simulink model "TractionEmotorSoftwareArch_DataBus"  (R2026a)
settings: Solver=FixedStepDiscrete
settings Model: DataDictionary=TractionEmotorSoftwareArchInterfaceData.sldd  EnableAccessToBaseWorkspace=off  OrderFunctionsByDependency=on  Creator=dakaihu  LastModifiedBy=dakaihu

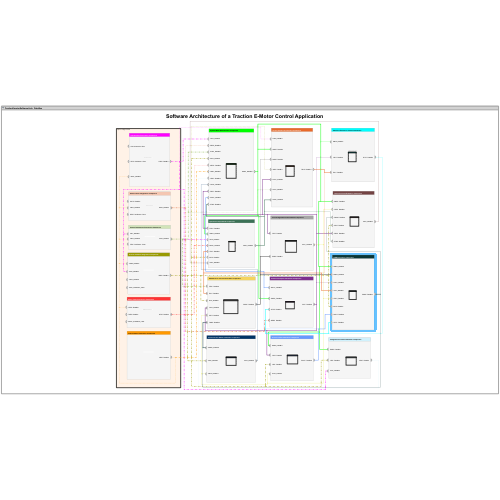
[thumbnail: Simulink's stored preview of the top-level diagram]
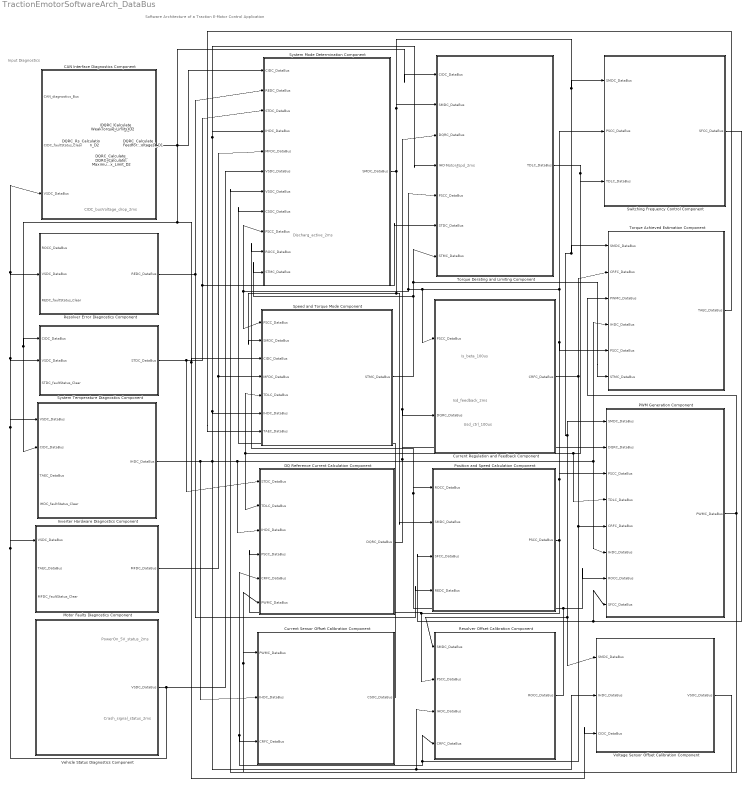
== system TractionEmotorSoftwareArch_DataBus ==
  note: Motor_spd_2ms
  note: Crash_signal_status_2ms
  note: PowerOn_5V_status_2ms
  note: Discharg_active_2ms
  note: Usd_ctrl_100us
  note: Isd_feedback_2ms
  note: Is_beta_100us
  note: CIDC_busVoltage_drop_2ms
  note: Input Diagnostics
  note: Software Architecture of a Traction E-Motor Control Application
  DQRC_Calculate_Feedforward_Voltages _D1 : Inport  OutputFunctionCall=on
  DQRC_Calculate_Optimal_Flux_D1 : Inport  Port=2  OutputFunctionCall=on
  DQRC_Flux_Weakening_Control_D1 : Inport  Port=3  OutputFunctionCall=on
  DQRC_Rs_Calculation_D2 : Inport  Port=4  OutputFunctionCall=on
  DQRC_Calculate_Maximum_Flux_Limit_D2 : Inport  Port=5  OutputFunctionCall=on
  DQRC_Calculate_Torque_Limits_D2 : Inport  Port=6  OutputFunctionCall=on
  CAN Interface Diagnostics Component : Subsystem
      settings: PortSchema="{\"entries\":[{\"content\":{\"headerSize\":26,\"margin\":15,\"minimumSpacing\":25,\"sides\":[{\"content\":{\"connectorIds\":[\"In2\",\"In1\",\"In3\"]},\"type\":\"ConnectorPlacement.EquallySpacedRectSide\",\"uuid\":\"3a2e990d-2ce1-4c6a-a08e-49004fced93c\"},{\"content\":{\"connectorIds\":[\"Out1\"],\"side\":\"RIGHT\"},\"type\":\"ConnectorPlacement.EquallySpacedRectSide\",\"uuid\":\"2e4f52de-0426-461f-b804-44573dbe364d\"},{\"content\":{\"connectorIds\":[],\"side\":\"TOP\"},\"type\":\"ConnectorPlacement.EquallySpacedRectSide\",\"uuid\":\"accbd54d-36a1-4bba-b227-ea03e90f0849\"}]},\"type\":\"ConnectorPlacement.EquallySpacedConnector\",\"uuid\":\"703f56ad-5037-4d99-b3d7-1bfb32b6a309\"}],\"packageUris\":[\"http://schema.mathworks.com/mf0/Connector/R2020b\"],\"version\":\"1.0\"}"
  "Current Regulation and Feedback Component " : Subsystem
      settings: PortSchema="{\"entries\":[{\"content\":{\"headerSize\":26,\"margin\":15,\"minimumSpacing\":25,\"sides\":[{\"content\":{\"connectorIds\":[\"In1\",\"In2\"]},\"type\":\"ConnectorPlacement.EquallySpacedRectSide\",\"uuid\":\"a71464e4-ef65-4500-8253-61f4bcbf30c4\"},{\"content\":{\"connectorIds\":[\"Out1\"],\"side\":\"RIGHT\"},\"type\":\"ConnectorPlacement.EquallySpacedRectSide\",\"uuid\":\"1bcf2d4f-45fa-4d52-8581-70b7b3dbffa8\"},{\"content\":{\"connectorIds\":[],\"side\":\"TOP\"},\"type\":\"ConnectorPlacement.EquallySpacedRectSide\",\"uuid\":\"1184bab8-6b51-4118-818c-c187fd989a95\"},{\"content\":{\"connectorIds\":[],\"side\":\"HIDDEN\"},\"type\":\"ConnectorPlacement.EquallySpacedRectSide\",\"uuid\":\"65ee186c-6391-47f9-9292-b3d987265f69\"}]},\"type\":\"ConnectorPlacement.EquallySpacedConnector\",\"uuid\":\"052954ad-d64a-4fb3-8bba-30843ae03591\"}],\"packageUris\":[\"http://schema.mathworks.com/mf0/Connector/R2020b\"],\"version\":\"1.0\"}"
  "Current Sensor Offset Calibration Component " : Subsystem
      settings: PortSchema="{\"entries\":[{\"content\":{\"headerSize\":26,\"margin\":15,\"minimumSpacing\":25,\"sides\":[{\"content\":{\"connectorIds\":[\"In1\",\"In2\",\"In3\"]},\"type\":\"ConnectorPlacement.EquallySpacedRectSide\",\"uuid\":\"a71464e4-ef65-4500-8253-61f4bcbf30c4\"},{\"content\":{\"connectorIds\":[\"Out1\"],\"side\":\"RIGHT\"},\"type\":\"ConnectorPlacement.EquallySpacedRectSide\",\"uuid\":\"1bcf2d4f-45fa-4d52-8581-70b7b3dbffa8\"},{\"content\":{\"connectorIds\":[],\"side\":\"TOP\"},\"type\":\"ConnectorPlacement.EquallySpacedRectSide\",\"uuid\":\"1184bab8-6b51-4118-818c-c187fd989a95\"},{\"content\":{\"connectorIds\":[],\"side\":\"HIDDEN\"},\"type\":\"ConnectorPlacement.EquallySpacedRectSide\",\"uuid\":\"65ee186c-6391-47f9-9292-b3d987265f69\"}]},\"type\":\"ConnectorPlacement.EquallySpacedConnector\",\"uuid\":\"052954ad-d64a-4fb3-8bba-30843ae03591\"}],\"packageUris\":[\"http://schema.mathworks.com/mf0/Connector/R2020b\"],\"version\":\"1.0\"}"
  DQ Reference Current Calculation Component : Subsystem
      settings: PortSchema="{\"entries\":[{\"content\":{\"headerSize\":26,\"margin\":15,\"minimumSpacing\":25,\"sides\":[{\"content\":{\"connectorIds\":[\"In1\",\"In2\",\"In6\",\"In3\",\"In4\",\"In5\"]},\"type\":\"ConnectorPlacement.EquallySpacedRectSide\",\"uuid\":\"a71464e4-ef65-4500-8253-61f4bcbf30c4\"},{\"content\":{\"connectorIds\":[\"Out1\"],\"side\":\"RIGHT\"},\"type\":\"ConnectorPlacement.EquallySpacedRectSide\",\"uuid\":\"1bcf2d4f-45fa-4d52-8581-70b7b3dbffa8\"},{\"content\":{\"connectorIds\":[],\"side\":\"TOP\"},\"type\":\"ConnectorPlacement.EquallySpacedRectSide\",\"uuid\":\"1184bab8-6b51-4118-818c-c187fd989a95\"},{\"content\":{\"connectorIds\":[],\"side\":\"HIDDEN\"},\"type\":\"ConnectorPlacement.EquallySpacedRectSide\",\"uuid\":\"65ee186c-6391-47f9-9292-b3d987265f69\"}]},\"type\":\"ConnectorPlacement.EquallySpacedConnector\",\"uuid\":\"052954ad-d64a-4fb3-8bba-30843ae03591\"}],\"packageUris\":[\"http://schema.mathworks.com/mf0/Connector/R2020b\"],\"version\":\"1.0\"}"
  Inverter Hardware Diagnostics Component : Subsystem
      settings: PortSchema="{\"entries\":[{\"content\":{\"headerSize\":26,\"margin\":15,\"minimumSpacing\":25,\"sides\":[{\"content\":{\"connectorIds\":[\"In1\",\"In2\",\"In3\",\"In4\"]},\"type\":\"ConnectorPlacement.EquallySpacedRectSide\",\"uuid\":\"3a2e990d-2ce1-4c6a-a08e-49004fced93c\"},{\"content\":{\"connectorIds\":[\"Out1\"],\"side\":\"RIGHT\"},\"type\":\"ConnectorPlacement.EquallySpacedRectSide\",\"uuid\":\"2e4f52de-0426-461f-b804-44573dbe364d\"},{\"content\":{\"connectorIds\":[],\"side\":\"TOP\"},\"type\":\"ConnectorPlacement.EquallySpacedRectSide\",\"uuid\":\"accbd54d-36a1-4bba-b227-ea03e90f0849\"}]},\"type\":\"ConnectorPlacement.EquallySpacedConnector\",\"uuid\":\"703f56ad-5037-4d99-b3d7-1bfb32b6a309\"}],\"packageUris\":[\"http://schema.mathworks.com/mf0/Connector/R2020b\"],\"version\":\"1.0\"}"
  Motor Faults Diagnostics Component : Subsystem
      settings: PortSchema="{\"entries\":[{\"content\":{\"headerSize\":26,\"margin\":15,\"minimumSpacing\":25,\"sides\":[{\"content\":{\"connectorIds\":[\"In1\",\"In2\",\"In3\"]},\"type\":\"ConnectorPlacement.EquallySpacedRectSide\",\"uuid\":\"3a2e990d-2ce1-4c6a-a08e-49004fced93c\"},{\"content\":{\"connectorIds\":[\"Out1\"],\"side\":\"RIGHT\"},\"type\":\"ConnectorPlacement.EquallySpacedRectSide\",\"uuid\":\"2e4f52de-0426-461f-b804-44573dbe364d\"},{\"content\":{\"connectorIds\":[],\"side\":\"TOP\"},\"type\":\"ConnectorPlacement.EquallySpacedRectSide\",\"uuid\":\"accbd54d-36a1-4bba-b227-ea03e90f0849\"}]},\"type\":\"ConnectorPlacement.EquallySpacedConnector\",\"uuid\":\"703f56ad-5037-4d99-b3d7-1bfb32b6a309\"}],\"packageUris\":[\"http://schema.mathworks.com/mf0/Connector/R2020b\"],\"version\":\"1.0\"}"
  PWM Generation Component : Subsystem
      settings: PortSchema="{\"entries\":[{\"content\":{\"headerSize\":26,\"margin\":15,\"minimumSpacing\":25,\"sides\":[{\"content\":{\"connectorIds\":[\"In2\",\"In1\",\"In3\",\"In4\",\"In6\",\"In7\",\"In8\",\"In5\"]},\"type\":\"ConnectorPlacement.EquallySpacedRectSide\",\"uuid\":\"a71464e4-ef65-4500-8253-61f4bcbf30c4\"},{\"content\":{\"connectorIds\":[\"Out1\"],\"side\":\"RIGHT\"},\"type\":\"ConnectorPlacement.EquallySpacedRectSide\",\"uuid\":\"1bcf2d4f-45fa-4d52-8581-70b7b3dbffa8\"},{\"content\":{\"connectorIds\":[],\"side\":\"TOP\"},\"type\":\"ConnectorPlacement.EquallySpacedRectSide\",\"uuid\":\"1184bab8-6b51-4118-818c-c187fd989a95\"},{\"content\":{\"connectorIds\":[],\"side\":\"HIDDEN\"},\"type\":\"ConnectorPlacement.EquallySpacedRectSide\",\"uuid\":\"65ee186c-6391-47f9-9292-b3d987265f69\"}]},\"type\":\"ConnectorPlacement.EquallySpacedConnector\",\"uuid\":\"052954ad-d64a-4fb3-8bba-30843ae03591\"}],\"packageUris\":[\"http://schema.mathworks.com/mf0/Connector/R2020b\"],\"version\":\"1.0\"}"
  Position and Speed Calculation Component : Subsystem
      settings: PortSchema="{\"entries\":[{\"content\":{\"headerSize\":26,\"margin\":15,\"minimumSpacing\":25,\"sides\":[{\"content\":{\"connectorIds\":[\"In1\",\"In2\",\"In3\",\"In4\"]},\"type\":\"ConnectorPlacement.EquallySpacedRectSide\",\"uuid\":\"a71464e4-ef65-4500-8253-61f4bcbf30c4\"},{\"content\":{\"connectorIds\":[\"Out1\"],\"side\":\"RIGHT\"},\"type\":\"ConnectorPlacement.EquallySpacedRectSide\",\"uuid\":\"1bcf2d4f-45fa-4d52-8581-70b7b3dbffa8\"},{\"content\":{\"connectorIds\":[],\"side\":\"TOP\"},\"type\":\"ConnectorPlacement.EquallySpacedRectSide\",\"uuid\":\"1184bab8-6b51-4118-818c-c187fd989a95\"},{\"content\":{\"connectorIds\":[],\"side\":\"HIDDEN\"},\"type\":\"ConnectorPlacement.EquallySpacedRectSide\",\"uuid\":\"65ee186c-6391-47f9-9292-b3d987265f69\"}]},\"type\":\"ConnectorPlacement.EquallySpacedConnector\",\"uuid\":\"052954ad-d64a-4fb3-8bba-30843ae03591\"}],\"packageUris\":[\"http://schema.mathworks.com/mf0/Connector/R2020b\"],\"version\":\"1.0\"}"
  Resolver Error Diagnostics Component : Subsystem
      settings: PortSchema="{\"entries\":[{\"content\":{\"headerSize\":26,\"margin\":15,\"minimumSpacing\":25,\"sides\":[{\"content\":{\"connectorIds\":[\"In1\",\"In2\",\"In3\"]},\"type\":\"ConnectorPlacement.EquallySpacedRectSide\",\"uuid\":\"3a2e990d-2ce1-4c6a-a08e-49004fced93c\"},{\"content\":{\"connectorIds\":[\"Out1\"],\"side\":\"RIGHT\"},\"type\":\"ConnectorPlacement.EquallySpacedRectSide\",\"uuid\":\"2e4f52de-0426-461f-b804-44573dbe364d\"},{\"content\":{\"side\":\"TOP\"},\"type\":\"ConnectorPlacement.EquallySpacedRectSide\",\"uuid\":\"accbd54d-36a1-4bba-b227-ea03e90f0849\"}]},\"type\":\"ConnectorPlacement.EquallySpacedConnector\",\"uuid\":\"703f56ad-5037-4d99-b3d7-1bfb32b6a309\"}],\"packageUris\":[\"http://schema.mathworks.com/mf0/Connector/R2020b\"],\"version\":\"1.0\"}"
  "Resolver Offset Calibration Component " : Subsystem
      settings: PortSchema="{\"entries\":[{\"content\":{\"headerSize\":26,\"margin\":15,\"minimumSpacing\":25,\"sides\":[{\"content\":{\"connectorIds\":[\"In1\",\"In2\",\"In3\",\"In4\"]},\"type\":\"ConnectorPlacement.EquallySpacedRectSide\",\"uuid\":\"b2f30fca-3d8e-46ee-af1d-282b22b9b844\"},{\"content\":{\"connectorIds\":[\"Out1\"],\"side\":\"RIGHT\"},\"type\":\"ConnectorPlacement.EquallySpacedRectSide\",\"uuid\":\"2d7d706d-eac4-4c73-84e8-2a36a393a616\"},{\"content\":{\"connectorIds\":[],\"side\":\"TOP\"},\"type\":\"ConnectorPlacement.EquallySpacedRectSide\",\"uuid\":\"b52ae510-b7cc-4ed0-8d34-4a095deae41b\"}]},\"type\":\"ConnectorPlacement.EquallySpacedConnector\",\"uuid\":\"1257e7cc-1858-4bc4-ab05-7b00060cf0d5\"}],\"packageUris\":[\"http://schema.mathworks.com/mf0/Connector/R2020b\"],\"version\":\"1.0\"}"
  Speed and Torque Mode Component : Subsystem
      settings: PortSchema="{\"entries\":[{\"content\":{\"headerSize\":26,\"margin\":15,\"minimumSpacing\":25,\"sides\":[{\"content\":{\"connectorIds\":[\"In4\",\"In1\",\"In2\",\"In3\",\"In5\",\"In7\",\"In6\"]},\"type\":\"ConnectorPlacement.EquallySpacedRectSide\",\"uuid\":\"a71464e4-ef65-4500-8253-61f4bcbf30c4\"},{\"content\":{\"connectorIds\":[\"Out1\"],\"side\":\"RIGHT\"},\"type\":\"ConnectorPlacement.EquallySpacedRectSide\",\"uuid\":\"1bcf2d4f-45fa-4d52-8581-70b7b3dbffa8\"},{\"content\":{\"connectorIds\":[],\"side\":\"TOP\"},\"type\":\"ConnectorPlacement.EquallySpacedRectSide\",\"uuid\":\"1184bab8-6b51-4118-818c-c187fd989a95\"},{\"content\":{\"connectorIds\":[],\"side\":\"HIDDEN\"},\"type\":\"ConnectorPlacement.EquallySpacedRectSide\",\"uuid\":\"65ee186c-6391-47f9-9292-b3d987265f69\"}]},\"type\":\"ConnectorPlacement.EquallySpacedConnector\",\"uuid\":\"052954ad-d64a-4fb3-8bba-30843ae03591\"}],\"packageUris\":[\"http://schema.mathworks.com/mf0/Connector/R2020b\"],\"version\":\"1.0\"}"
  Switching Frequency Control Component : Subsystem
      settings: PortSchema="{\"entries\":[{\"content\":{\"headerSize\":26,\"margin\":15,\"minimumSpacing\":25,\"sides\":[{\"content\":{\"connectorIds\":[\"In1\",\"In2\",\"In3\"]},\"type\":\"ConnectorPlacement.EquallySpacedRectSide\",\"uuid\":\"a71464e4-ef65-4500-8253-61f4bcbf30c4\"},{\"content\":{\"connectorIds\":[\"Out1\"],\"side\":\"RIGHT\"},\"type\":\"ConnectorPlacement.EquallySpacedRectSide\",\"uuid\":\"1bcf2d4f-45fa-4d52-8581-70b7b3dbffa8\"},{\"content\":{\"connectorIds\":[],\"side\":\"TOP\"},\"type\":\"ConnectorPlacement.EquallySpacedRectSide\",\"uuid\":\"1184bab8-6b51-4118-818c-c187fd989a95\"},{\"content\":{\"connectorIds\":[],\"side\":\"HIDDEN\"},\"type\":\"ConnectorPlacement.EquallySpacedRectSide\",\"uuid\":\"65ee186c-6391-47f9-9292-b3d987265f69\"}]},\"type\":\"ConnectorPlacement.EquallySpacedConnector\",\"uuid\":\"052954ad-d64a-4fb3-8bba-30843ae03591\"}],\"packageUris\":[\"http://schema.mathworks.com/mf0/Connector/R2020b\"],\"version\":\"1.0\"}"
  "System Mode Determination Component " : Subsystem
      settings: PortSchema="{\"entries\":[{\"content\":{\"headerSize\":26,\"margin\":15,\"minimumSpacing\":25,\"sides\":[{\"content\":{\"connectorIds\":[\"In1\",\"In2\",\"In3\",\"In4\",\"In5\",\"In6\",\"In9\",\"In8\",\"In10\",\"In7\",\"In11\"]},\"type\":\"ConnectorPlacement.EquallySpacedRectSide\",\"uuid\":\"a71464e4-ef65-4500-8253-61f4bcbf30c4\"},{\"content\":{\"connectorIds\":[\"Out1\"],\"side\":\"RIGHT\"},\"type\":\"ConnectorPlacement.EquallySpacedRectSide\",\"uuid\":\"1bcf2d4f-45fa-4d52-8581-70b7b3dbffa8\"},{\"content\":{\"connectorIds\":[],\"side\":\"TOP\"},\"type\":\"ConnectorPlacement.EquallySpacedRectSide\",\"uuid\":\"1184bab8-6b51-4118-818c-c187fd989a95\"},{\"content\":{\"connectorIds\":[],\"side\":\"BOTTOM\"},\"type\":\"ConnectorPlacement.EquallySpacedRectSide\",\"uuid\":\"db64044a-7d50-4610-bfd1-d03b668d605f\"},{\"content\":{\"connectorIds\":[],\"side\":\"HIDDEN\"},\"type\":\"ConnectorPlacement.EquallySpacedRectSide\",\"uuid\":\"65ee186c-6391-47f9-9292-b3d987265f69\"}]},\"type\":\"ConnectorPlacement.EquallySpacedConnector\",\"uuid\":\"052954ad-d64a-4fb3-8bba-30843ae03591\"}],\"packageUris\":[\"http://schema.mathworks.com/mf0/Connector/R2020b\"],\"version\":\"1.0\"}"
  System Temperature Diagnostics Component : Subsystem
      settings: PortSchema="{\"entries\":[{\"content\":{\"headerSize\":26,\"margin\":15,\"minimumSpacing\":25,\"sides\":[{\"content\":{\"connectorIds\":[\"In1\",\"In2\",\"In3\"]},\"type\":\"ConnectorPlacement.EquallySpacedRectSide\",\"uuid\":\"3a2e990d-2ce1-4c6a-a08e-49004fced93c\"},{\"content\":{\"connectorIds\":[\"Out1\"],\"side\":\"RIGHT\"},\"type\":\"ConnectorPlacement.EquallySpacedRectSide\",\"uuid\":\"2e4f52de-0426-461f-b804-44573dbe364d\"},{\"content\":{\"connectorIds\":[],\"side\":\"TOP\"},\"type\":\"ConnectorPlacement.EquallySpacedRectSide\",\"uuid\":\"accbd54d-36a1-4bba-b227-ea03e90f0849\"}]},\"type\":\"ConnectorPlacement.EquallySpacedConnector\",\"uuid\":\"703f56ad-5037-4d99-b3d7-1bfb32b6a309\"}],\"packageUris\":[\"http://schema.mathworks.com/mf0/Connector/R2020b\"],\"version\":\"1.0\"}"
  Torque Achieved Estimation Component : Subsystem
      settings: PortSchema="{\"entries\":[{\"content\":{\"headerSize\":26,\"margin\":15,\"minimumSpacing\":25,\"sides\":[{\"content\":{\"connectorIds\":[\"In1\",\"In2\",\"In3\",\"In4\",\"In5\",\"In6\"]},\"type\":\"ConnectorPlacement.EquallySpacedRectSide\",\"uuid\":\"a71464e4-ef65-4500-8253-61f4bcbf30c4\"},{\"content\":{\"connectorIds\":[\"Out1\"],\"side\":\"RIGHT\"},\"type\":\"ConnectorPlacement.EquallySpacedRectSide\",\"uuid\":\"1bcf2d4f-45fa-4d52-8581-70b7b3dbffa8\"},{\"content\":{\"connectorIds\":[],\"side\":\"TOP\"},\"type\":\"ConnectorPlacement.EquallySpacedRectSide\",\"uuid\":\"1184bab8-6b51-4118-818c-c187fd989a95\"},{\"content\":{\"connectorIds\":[],\"side\":\"HIDDEN\"},\"type\":\"ConnectorPlacement.EquallySpacedRectSide\",\"uuid\":\"65ee186c-6391-47f9-9292-b3d987265f69\"}]},\"type\":\"ConnectorPlacement.EquallySpacedConnector\",\"uuid\":\"052954ad-d64a-4fb3-8bba-30843ae03591\"}],\"packageUris\":[\"http://schema.mathworks.com/mf0/Connector/R2020b\"],\"version\":\"1.0\"}"
  Torque Derating and Limiting Component : Subsystem
      settings: PortSchema="{\"entries\":[{\"content\":{\"headerSize\":26,\"margin\":15,\"minimumSpacing\":25,\"sides\":[{\"content\":{\"connectorIds\":[\"In5\",\"In1\",\"In2\",\"In3\",\"In4\",\"In6\",\"In7\"]},\"type\":\"ConnectorPlacement.EquallySpacedRectSide\",\"uuid\":\"fd31d295-2ee8-4010-a085-72a956fb88db\"},{\"content\":{\"connectorIds\":[\"Out1\"],\"side\":\"RIGHT\"},\"type\":\"ConnectorPlacement.EquallySpacedRectSide\",\"uuid\":\"6e15e65a-8b2c-4657-b6d9-6871ed377dcc\"},{\"content\":{\"connectorIds\":[],\"side\":\"TOP\"},\"type\":\"ConnectorPlacement.EquallySpacedRectSide\",\"uuid\":\"e10f5a11-10a3-425e-91ff-fff14d159c09\"},{\"content\":{\"connectorIds\":[],\"side\":\"BOTTOM\"},\"type\":\"ConnectorPlacement.EquallySpacedRectSide\",\"uuid\":\"618ca321-1f5f-4aa6-a247-3a346143f509\"}]},\"type\":\"ConnectorPlacement.EquallySpacedConnector\",\"uuid\":\"062b7cf1-4df3-4671-ab85-e62a20780700\"}],\"packageUris\":[\"http://schema.mathworks.com/mf0/Connector/R2020b\"],\"version\":\"1.0\"}"
  Vehicle Status Diagnostics Component : Subsystem
      settings: PortSchema="{\"entries\":[{\"content\":{\"headerSize\":26,\"margin\":15,\"minimumSpacing\":25,\"sides\":[{\"content\":{\"connectorIds\":[]},\"type\":\"ConnectorPlacement.EquallySpacedRectSide\",\"uuid\":\"3a2e990d-2ce1-4c6a-a08e-49004fced93c\"},{\"content\":{\"connectorIds\":[\"Out1\"],\"side\":\"RIGHT\"},\"type\":\"ConnectorPlacement.EquallySpacedRectSide\",\"uuid\":\"2e4f52de-0426-461f-b804-44573dbe364d\"},{\"content\":{\"connectorIds\":[],\"side\":\"TOP\"},\"type\":\"ConnectorPlacement.EquallySpacedRectSide\",\"uuid\":\"accbd54d-36a1-4bba-b227-ea03e90f0849\"}]},\"type\":\"ConnectorPlacement.EquallySpacedConnector\",\"uuid\":\"703f56ad-5037-4d99-b3d7-1bfb32b6a309\"}],\"packageUris\":[\"http://schema.mathworks.com/mf0/Connector/R2020b\"],\"version\":\"1.0\"}"
  Voltage Sensor Offset Calibration Component : Subsystem
      settings: PortSchema="{\"entries\":[{\"content\":{\"headerSize\":26,\"margin\":15,\"minimumSpacing\":25,\"sides\":[{\"content\":{\"connectorIds\":[\"In1\",\"In3\",\"In2\"]},\"type\":\"ConnectorPlacement.EquallySpacedRectSide\",\"uuid\":\"a71464e4-ef65-4500-8253-61f4bcbf30c4\"},{\"content\":{\"connectorIds\":[\"Out1\"],\"side\":\"RIGHT\"},\"type\":\"ConnectorPlacement.EquallySpacedRectSide\",\"uuid\":\"1bcf2d4f-45fa-4d52-8581-70b7b3dbffa8\"},{\"content\":{\"connectorIds\":[],\"side\":\"TOP\"},\"type\":\"ConnectorPlacement.EquallySpacedRectSide\",\"uuid\":\"1184bab8-6b51-4118-818c-c187fd989a95\"},{\"content\":{\"connectorIds\":[],\"side\":\"HIDDEN\"},\"type\":\"ConnectorPlacement.EquallySpacedRectSide\",\"uuid\":\"65ee186c-6391-47f9-9292-b3d987265f69\"}]},\"type\":\"ConnectorPlacement.EquallySpacedConnector\",\"uuid\":\"052954ad-d64a-4fb3-8bba-30843ae03591\"}],\"packageUris\":[\"http://schema.mathworks.com/mf0/Connector/R2020b\"],\"version\":\"1.0\"}"
  wires:
  Resolver Error Diagnostics Component/1(REDC_DataBus) -> "System Mode Determination Component "/2(REDC_DataBus), Position and Speed Calculation Component/4(REDC_DataBus)
  System Temperature Diagnostics Component/1(STDC_DataBus) -> DQ Reference Current Calculation Component/1(STDC_DataBus), Torque Derating and Limiting Component/6(STDC_DataBus), "System Mode Determination Component "/3(STDC_DataBus)
  Inverter Hardware Diagnostics Component/1(IHDC_DataBus) -> "Current Sensor Offset Calibration Component "/2(IHDC_DataBus), PWM Generation Component/7(IHDC_DataBus), Torque Achieved Estimation Component/4(IHDC_DataBus), DQ Reference Current Calculation Component/6(IHDC_DataBus), "Resolver Offset Calibration Component "/3(IHDC_DataBus), Voltage Sensor Offset Calibration Component/3(IHDC_DataBus), "System Mode Determination Component "/4(IHDC_DataBus), Torque Derating and Limiting Component/3(IHDC_DataBus), Speed and Torque Mode Component/7(IHDC_DataBus)
  Motor Faults Diagnostics Component/1(MFDC_DataBus) -> "System Mode Determination Component "/5(MFDC_DataBus), Speed and Torque Mode Component/3(MFDC_DataBus)
  Vehicle Status Diagnostics Component/1(VSDC_DataBus) -> "System Mode Determination Component "/6(VSDC_DataBus), Motor Faults Diagnostics Component/1(VSDC_DataBus), System Temperature Diagnostics Component/2(VSDC_DataBus), Resolver Error Diagnostics Component/2(VSDC_DataBus), CAN Interface Diagnostics Component/3(VSDC_DataBus), Inverter Hardware Diagnostics Component/1(VSDC_DataBus)
  "System Mode Determination Component "/1(SMDC_DataBus) -> Position and Speed Calculation Component/2(SMDC_DataBus), Speed and Torque Mode Component/1(SMDC_DataBus), Torque Derating and Limiting Component/1(SMDC_DataBus), PWM Generation Component/2(SMDC_DataBus), Voltage Sensor Offset Calibration Component/1(SMDC_DataBus), "Resolver Offset Calibration Component "/1(SMDC_DataBus), Torque Achieved Estimation Component/1(SMDC_DataBus), Switching Frequency Control Component/1(SMDC_DataBus)
  "Resolver Offset Calibration Component "/1(ROCC_DataBus) -> "System Mode Determination Component "/7(ROCC_DataBus), Position and Speed Calculation Component/1(ROCC_DataBus), PWM Generation Component/8(ROCC_DataBus)
  "Current Sensor Offset Calibration Component "/1(CSOC_DataBus) -> "System Mode Determination Component "/8(CSOC_DataBus)
  Voltage Sensor Offset Calibration Component/1(VSOC_DataBus) -> "System Mode Determination Component "/9(VSOC_DataBus)
  Position and Speed Calculation Component/1(PSCC_DataBus) -> Torque Achieved Estimation Component/5(PSCC_DataBus), "Current Regulation and Feedback Component "/1(PSCC_DataBus), Torque Derating and Limiting Component/4(PSCC_DataBus), Speed and Torque Mode Component/4(PSCC_DataBus), "System Mode Determination Component "/10(PSCC_DataBus), Switching Frequency Control Component/2(PSCC_DataBus), PWM Generation Component/3(PSCC_DataBus), "Resolver Offset Calibration Component "/2(PSCC_DataBus), DQ Reference Current Calculation Component/3(PSCC_DataBus)
  Speed and Torque Mode Component/1(STMC_DataBus) -> Torque Achieved Estimation Component/6(STMC_DataBus), Torque Derating and Limiting Component/7(STMC_DataBus), "System Mode Determination Component "/11(STMC_DataBus)
  DQ Reference Current Calculation Component/1(DQRC_DataBus) -> Torque Derating and Limiting Component/2(DQRC_DataBus), "Current Regulation and Feedback Component "/2(DQRC_DataBus), PWM Generation Component/1(DQRC_DataBus)
  Torque Derating and Limiting Component/1(TDLC_DataBus) -> Switching Frequency Control Component/3(TDLC_DataBus), PWM Generation Component/4(TDLC_DataBus), DQ Reference Current Calculation Component/2(TDLC_DataBus), Speed and Torque Mode Component/5(TDLC_DataBus)
  "Current Regulation and Feedback Component "/1(CRFC_DataBus) -> Torque Achieved Estimation Component/2(CRFC_DataBus), "Resolver Offset Calibration Component "/4(CRFC_DataBus), "Current Sensor Offset Calibration Component "/3(CRFC_DataBus), DQ Reference Current Calculation Component/4(CRFC_DataBus), PWM Generation Component/6(CRFC_DataBus)
  PWM Generation Component/1(PWMC_DataBus) -> DQ Reference Current Calculation Component/5(PWMC_DataBus), "Current Sensor Offset Calibration Component "/1(PWMC_DataBus), Torque Achieved Estimation Component/3(PWMC_DataBus)
  Switching Frequency Control Component/1(SFCC_DataBus) -> Position and Speed Calculation Component/3(SFCC_DataBus), PWM Generation Component/5(SFCC_DataBus)
  Torque Achieved Estimation Component/1(TAEC_DataBus) -> Speed and Torque Mode Component/6(TAEC_DataBus)
  CAN Interface Diagnostics Component/1(CIDC_DataBus) -> "System Mode Determination Component "/1(CIDC_DataBus), Speed and Torque Mode Component/2(CIDC_DataBus), Voltage Sensor Offset Calibration Component/2(CIDC_DataBus), Inverter Hardware Diagnostics Component/2(CIDC_DataBus), System Temperature Diagnostics Component/1(CIDC_DataBus), Torque Derating and Limiting Component/5(CIDC_DataBus)

== system TractionEmotorSoftwareArch_DataBus/CAN Interface Diagnostics Component ==
  note: CIDC: CAN Interface Diagnostics Component
  Bus Element In1 : Inport  PortName=CIDC_faultStatus_Clear
  Bus Element In2 : Inport  Port=2  PortName=CAN_diagnostics_Bus
  Bus Element In3 : Inport  Port=3  PortName=VSDC_DataBus
  Bus Element Out8 : Outport  PortName=CIDC_DataBus

== system TractionEmotorSoftwareArch_DataBus/Current Regulation and Feedback Component  ==
  note: CRFC: Currents Regulation and Feedback Component
  Bus Element In1 : Inport  PortName=PSCC_DataBus
  Bus Element In2 : Inport  Port=2  PortName=DQRC_DataBus
  CRFC : ModelReference  ModelNameDialog=CurrentRegulationandFeedbackComponent  SimulationMode=Normal  ScheduleRates=on  ModelReferenceVersion=7.0
      settings: PortSchema="{\"entries\":[{\"content\":{\"headerSize\":38,\"margin\":15,\"minimumSpacing\":25,\"sides\":[{\"content\":{\"connectorIds\":[\"In1\",\"In2\",\"In3\",\"In4\",\"In5\",\"In6\",\"In7\",\"In8\",\"In9\",\"In10\",\"In11\",\"In12\"]},\"type\":\"ConnectorPlacement.EquallySpacedRectSide\",\"uuid\":\"43f14977-22c5-403b-bcbc-53575b3aceee\"},{\"content\":{\"connectorIds\":[\"Out1\",\"Out2\",\"Out3\",\"Out4\",\"Out5\",\"Out6\",\"Out7\",\"Out8\",\"Out9\",\"Out10\",\"Out11\"],\"side\":\"RIGHT\"},\"type\":\"ConnectorPlacement.EquallySpacedRectSide\",\"uuid\":\"d93cf4b9-940c-436a-9f2b-9eb79a050f7a\"},{\"content\":{\"side\":\"TOP\"},\"type\":\"ConnectorPlacement.EquallySpacedRectSide\",\"uuid\":\"b3e7cb9e-f235-4106-b3bb-4ca948939197\"},{\"content\":{\"side\":\"HIDDEN\"},\"type\":\"ConnectorPlacement.EquallySpacedRectSide\",\"uuid\":\"291ccf75-5793-4f13-97ee-51f98f8a6b6f\"}]},\"type\":\"ConnectorPlacement.EquallySpacedConnector\",\"uuid\":\"a3b713dd-1bd4-4226-93ff-27d7db6c05ec\"}],\"packageUris\":[\"http://schema.mathworks.com/mf0/Connector/R2020b\"],\"version\":\"1.0\"}"
  Bus Element Out1 : Outport  PortName=CRFC_DataBus

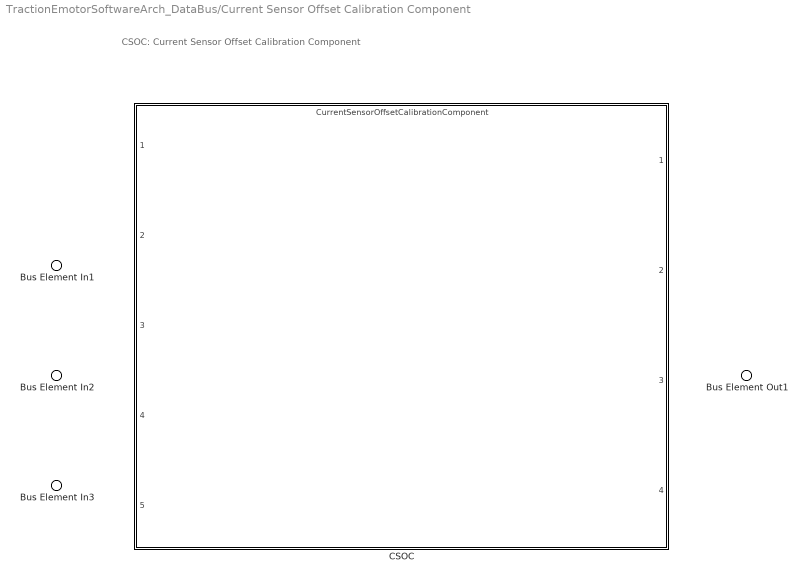
== system TractionEmotorSoftwareArch_DataBus/Current Sensor Offset Calibration Component  ==
  note: CSOC: Current Sensor Offset Calibration Component
  Bus Element In1 : Inport  PortName=PWMC_DataBus
  Bus Element In2 : Inport  Port=2  PortName=IHDC_DataBus
  Bus Element In3 : Inport  Port=3  PortName=CRFC_DataBus
  CSOC : ModelReference  ModelNameDialog=CurrentSensorOffsetCalibrationComponent  SimulationMode=Normal  ScheduleRates=on  ModelReferenceVersion=7.0
      settings: PortSchema="{\"entries\":[{\"content\":{\"headerSize\":38,\"margin\":15,\"minimumSpacing\":25,\"sides\":[{\"content\":{\"connectorIds\":[\"In1\",\"In2\",\"In3\",\"In4\",\"In5\"]},\"type\":\"ConnectorPlacement.EquallySpacedRectSide\",\"uuid\":\"43f14977-22c5-403b-bcbc-53575b3aceee\"},{\"content\":{\"connectorIds\":[\"Out1\",\"Out2\",\"Out3\",\"Out4\"],\"side\":\"RIGHT\"},\"type\":\"ConnectorPlacement.EquallySpacedRectSide\",\"uuid\":\"d93cf4b9-940c-436a-9f2b-9eb79a050f7a\"},{\"content\":{\"side\":\"TOP\"},\"type\":\"ConnectorPlacement.EquallySpacedRectSide\",\"uuid\":\"b3e7cb9e-f235-4106-b3bb-4ca948939197\"},{\"content\":{\"side\":\"HIDDEN\"},\"type\":\"ConnectorPlacement.EquallySpacedRectSide\",\"uuid\":\"d508bc3c-50c4-40a2-9dd3-c5ccc3c4a7e2\"}]},\"type\":\"ConnectorPlacement.EquallySpacedConnector\",\"uuid\":\"a3b713dd-1bd4-4226-93ff-27d7db6c05ec\"}],\"packageUris\":[\"http://schema.mathworks.com/mf0/Connector/R2020b\"],\"version\":\"1.0\"}"
  Bus Element Out1 : Outport  PortName=CSOC_DataBus

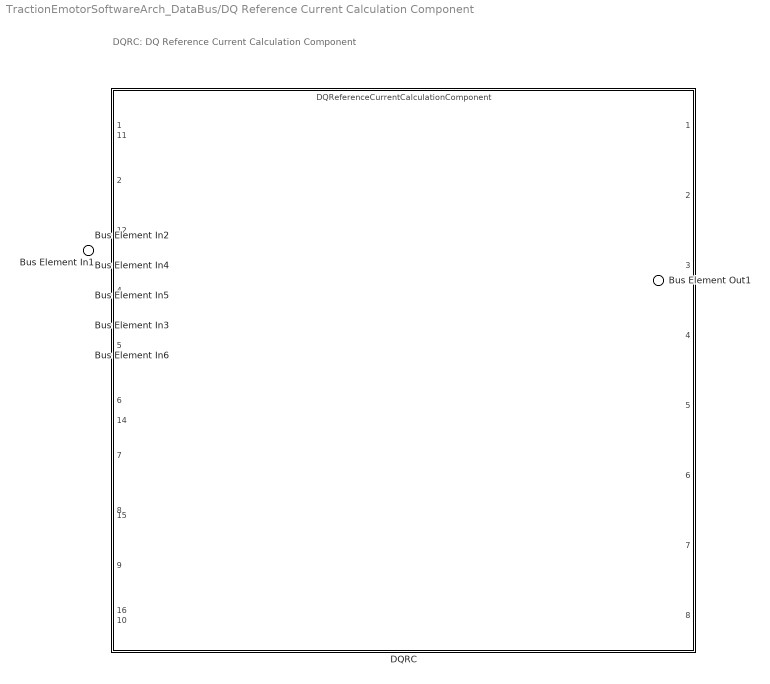
== system TractionEmotorSoftwareArch_DataBus/DQ Reference Current Calculation Component ==
  note: DQRC: DQ Reference Current Calculation Component
  Bus Element In1 : Inport  PortName=STDC_DataBus  Element=STDC_motorTemp_2ms
  Bus Element In2 : Inport  Port=2  PortName=TDLC_DataBus
  Bus Element In4 : Inport  Port=3  PortName=PSCC_DataBus
  Bus Element In5 : Inport  Port=4  PortName=CRFC_DataBus
  Bus Element In3 : Inport  Port=5  PortName=PWMC_DataBus
  Bus Element In6 : Inport  Port=6  PortName=IHDC_DataBus
  DQRC : ModelReference  ModelNameDialog=DQReferenceCurrentCalculationComponent  SimulationMode=Normal  ScheduleRates=on  ModelReferenceVersion=2.3
      settings: PortSchema="{\"entries\":[{\"content\":{\"headerSize\":38,\"margin\":15,\"minimumSpacing\":25,\"sides\":[{\"content\":{\"connectorIds\":[\"In1\",\"In2\",\"In3\",\"In4\",\"In5\",\"In6\",\"In7\",\"In8\",\"In9\",\"In10\"]},\"type\":\"ConnectorPlacement.EquallySpacedRectSide\",\"uuid\":\"43f14977-22c5-403b-bcbc-53575b3aceee\"},{\"content\":{\"connectorIds\":[\"Out1\",\"Out2\",\"Out3\",\"Out4\",\"Out5\",\"Out6\",\"Out7\",\"Out8\"],\"side\":\"RIGHT\"},\"type\":\"ConnectorPlacement.EquallySpacedRectSide\",\"uuid\":\"d93cf4b9-940c-436a-9f2b-9eb79a050f7a\"},{\"content\":{\"side\":\"TOP\"},\"type\":\"ConnectorPlacement.EquallySpacedRectSide\",\"uuid\":\"b3e7cb9e-f235-4106-b3bb-4ca948939197\"},{\"content\":{\"connectorIds\":[\"In11\",\"In12\",\"In13\",\"In14\",\"In15\",\"In16\"],\"side\":\"HIDDEN\"},\"type\":\"ConnectorPlacement.EquallySpacedRectSide\",\"uuid\":\"ecb0ba9f-b61e-4a54-9853-d15b952a8aaa\"}]},\"type\":\"ConnectorPlacement.EquallySpacedConnector\",\"uuid\":\"a3b713dd-1bd4-4226-93ff-27d7db6c05ec\"}],\"packageUris\":[\"http://schema.mathworks.com/mf0/Connector/R2020b\"],\"version\":\"1.0\"}"
  Bus Element Out1 : Outport  PortName=DQRC_DataBus

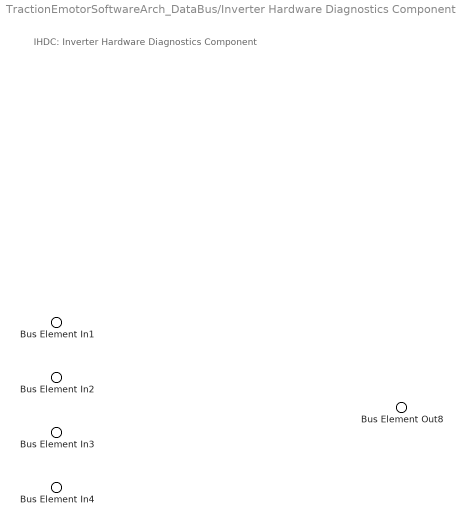
== system TractionEmotorSoftwareArch_DataBus/Inverter Hardware Diagnostics Component ==
  note: IHDC: Inverter Hardware Diagnostics Component
  Bus Element In1 : Inport  PortName=VSDC_DataBus
  Bus Element In2 : Inport  Port=2  PortName=CIDC_DataBus
  Bus Element In3 : Inport  Port=3  PortName=TAEC_DataBus
  Bus Element In4 : Inport  Port=4  PortName=IHDC_faultStatus_Clear
  Bus Element Out8 : Outport  PortName=IHDC_DataBus

== system TractionEmotorSoftwareArch_DataBus/Motor Faults Diagnostics Component ==
  note: MFDC: Motor Faults Diagnostics Component
  Bus Element In1 : Inport  PortName=VSDC_DataBus
  Bus Element In2 : Inport  Port=2  PortName=TAEC_DataBus
  Bus Element In3 : Inport  Port=3  PortName=MFDC_faultStatus_Clear
  Bus Element Out4 : Outport  PortName=MFDC_DataBus

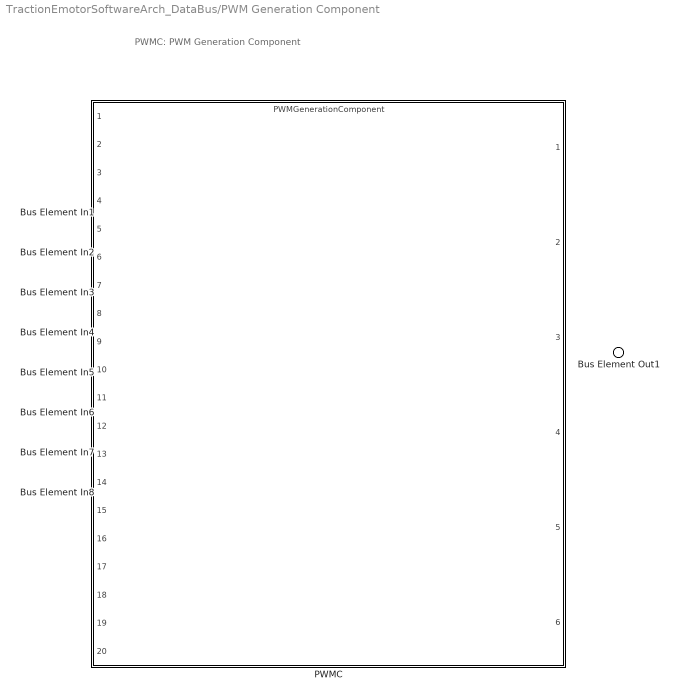
== system TractionEmotorSoftwareArch_DataBus/PWM Generation Component ==
  note: PWMC: PWM Generation Component
  Bus Element In1 : Inport  PortName=DQRC_DataBus
  Bus Element In2 : Inport  Port=2  PortName=SMDC_DataBus
  Bus Element In3 : Inport  Port=3  PortName=PSCC_DataBus
  Bus Element In4 : Inport  Port=4  PortName=TDLC_DataBus
  Bus Element In5 : Inport  Port=5  PortName=SFCC_DataBus
  Bus Element In6 : Inport  Port=6  PortName=CRFC_DataBus
  Bus Element In7 : Inport  Port=7  PortName=IHDC_DataBus
  Bus Element In8 : Inport  Port=8  PortName=ROCC_DataBus
  PWMC : ModelReference  ModelNameDialog=PWMGenerationComponent  SimulationMode=Normal  ScheduleRates=on  ModelReferenceVersion=7.0
      settings: PortSchema="{\"entries\":[{\"content\":{\"headerSize\":38,\"margin\":15,\"minimumSpacing\":25,\"sides\":[{\"content\":{\"connectorIds\":[\"In1\",\"In2\",\"In3\",\"In4\",\"In5\",\"In6\",\"In7\",\"In8\",\"In9\",\"In10\",\"In11\",\"In12\",\"In13\",\"In14\",\"In15\",\"In16\",\"In17\",\"In18\",\"In19\",\"In20\"]},\"type\":\"ConnectorPlacement.EquallySpacedRectSide\",\"uuid\":\"43f14977-22c5-403b-bcbc-53575b3aceee\"},{\"content\":{\"connectorIds\":[\"Out1\",\"Out2\",\"Out3\",\"Out4\",\"Out5\",\"Out6\"],\"side\":\"RIGHT\"},\"type\":\"ConnectorPlacement.EquallySpacedRectSide\",\"uuid\":\"d93cf4b9-940c-436a-9f2b-9eb79a050f7a\"},{\"content\":{\"side\":\"TOP\"},\"type\":\"ConnectorPlacement.EquallySpacedRectSide\",\"uuid\":\"b3e7cb9e-f235-4106-b3bb-4ca948939197\"},{\"content\":{\"side\":\"HIDDEN\"},\"type\":\"ConnectorPlacement.EquallySpacedRectSide\",\"uuid\":\"526cc332-2e45-43aa-9cbd-9944a0525fea\"}]},\"type\":\"ConnectorPlacement.EquallySpacedConnector\",\"uuid\":\"a3b713dd-1bd4-4226-93ff-27d7db6c05ec\"}],\"packageUris\":[\"http://schema.mathworks.com/mf0/Connector/R2020b\"],\"version\":\"1.0\"}"
  Bus Element Out1 : Outport  PortName=PWMC_DataBus

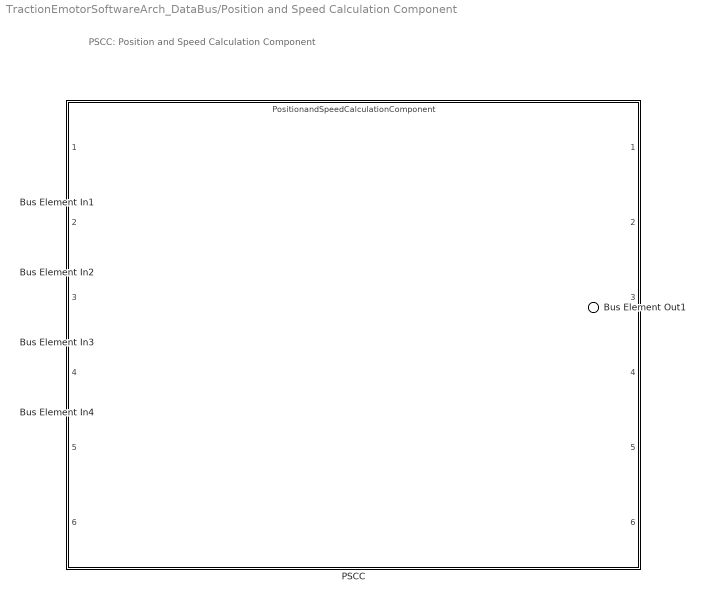
== system TractionEmotorSoftwareArch_DataBus/Position and Speed Calculation Component ==
  note: PSCC: Position and Speed Calculation Component
  Bus Element In1 : Inport  PortName=ROCC_DataBus
  Bus Element In2 : Inport  Port=2  PortName=SMDC_DataBus
  Bus Element In3 : Inport  Port=3  PortName=SFCC_DataBus
  Bus Element In4 : Inport  Port=4  PortName=REDC_DataBus
  PSCC : ModelReference  ModelNameDialog=PositionandSpeedCalculationComponent  SimulationMode=Normal  ScheduleRates=on  ModelReferenceVersion=7.0
      settings: PortSchema="{\"entries\":[{\"content\":{\"headerSize\":38,\"margin\":15,\"minimumSpacing\":25,\"sides\":[{\"content\":{\"connectorIds\":[\"In1\",\"In2\",\"In3\",\"In4\",\"In5\",\"In6\"]},\"type\":\"ConnectorPlacement.EquallySpacedRectSide\",\"uuid\":\"43f14977-22c5-403b-bcbc-53575b3aceee\"},{\"content\":{\"connectorIds\":[\"Out1\",\"Out2\",\"Out3\",\"Out4\",\"Out5\",\"Out6\"],\"side\":\"RIGHT\"},\"type\":\"ConnectorPlacement.EquallySpacedRectSide\",\"uuid\":\"d93cf4b9-940c-436a-9f2b-9eb79a050f7a\"},{\"content\":{\"side\":\"TOP\"},\"type\":\"ConnectorPlacement.EquallySpacedRectSide\",\"uuid\":\"b3e7cb9e-f235-4106-b3bb-4ca948939197\"},{\"content\":{\"side\":\"HIDDEN\"},\"type\":\"ConnectorPlacement.EquallySpacedRectSide\",\"uuid\":\"f9305b02-be4e-4f35-9a1b-e6cb4016013e\"}]},\"type\":\"ConnectorPlacement.EquallySpacedConnector\",\"uuid\":\"a3b713dd-1bd4-4226-93ff-27d7db6c05ec\"}],\"packageUris\":[\"http://schema.mathworks.com/mf0/Connector/R2020b\"],\"version\":\"1.0\"}"
  Bus Element Out1 : Outport  PortName=PSCC_DataBus

== system TractionEmotorSoftwareArch_DataBus/Resolver Error Diagnostics Component ==
  note: REDC: Resolver Error Diagnostics Component
  Bus Element In1 : Inport  PortName=ROCC_DataBus
  Bus Element In2 : Inport  Port=2  PortName=VSDC_DataBus
  Bus Element In3 : Inport  Port=3  PortName=REDC_faultStatus_Clear
  Bus Element Out1 : Outport  PortName=REDC_DataBus

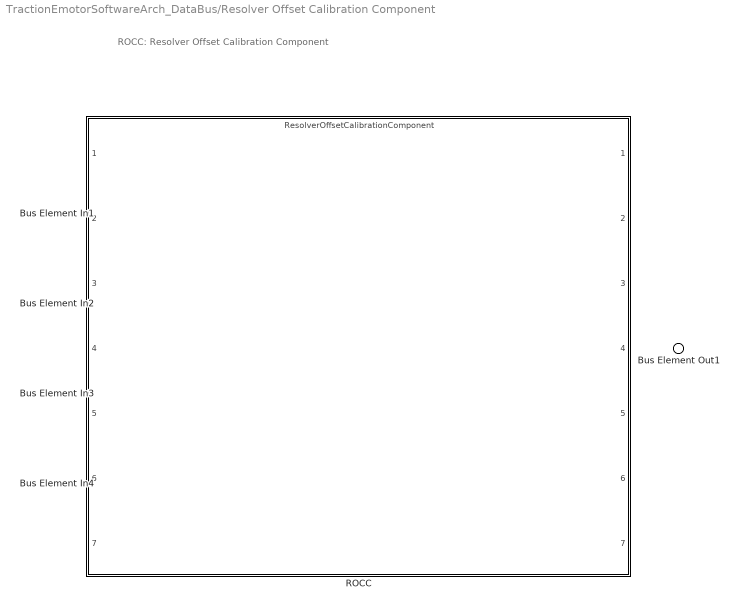
== system TractionEmotorSoftwareArch_DataBus/Resolver Offset Calibration Component  ==
  note: ROCC: Resolver Offset Calibration Component
  Bus Element In1 : Inport  PortName=SMDC_DataBus
  Bus Element In2 : Inport  Port=2  PortName=PSCC_DataBus
  Bus Element In3 : Inport  Port=3  PortName=IHDC_DataBus
  Bus Element In4 : Inport  Port=4  PortName=CRFC_DataBus
  ROCC : ModelReference  ModelNameDialog=ResolverOffsetCalibrationComponent  SimulationMode=Normal  ScheduleRates=on  ModelReferenceVersion=7.0
      settings: PortSchema="{\"entries\":[{\"content\":{\"headerSize\":38,\"margin\":15,\"minimumSpacing\":25,\"sides\":[{\"content\":{\"connectorIds\":[\"In1\",\"In2\",\"In3\",\"In4\",\"In5\",\"In6\",\"In7\"]},\"type\":\"ConnectorPlacement.EquallySpacedRectSide\",\"uuid\":\"43f14977-22c5-403b-bcbc-53575b3aceee\"},{\"content\":{\"connectorIds\":[\"Out1\",\"Out2\",\"Out3\",\"Out4\",\"Out5\",\"Out6\",\"Out7\"],\"side\":\"RIGHT\"},\"type\":\"ConnectorPlacement.EquallySpacedRectSide\",\"uuid\":\"d93cf4b9-940c-436a-9f2b-9eb79a050f7a\"},{\"content\":{\"side\":\"TOP\"},\"type\":\"ConnectorPlacement.EquallySpacedRectSide\",\"uuid\":\"b3e7cb9e-f235-4106-b3bb-4ca948939197\"},{\"content\":{\"side\":\"HIDDEN\"},\"type\":\"ConnectorPlacement.EquallySpacedRectSide\",\"uuid\":\"f515207f-401f-4fd2-a307-55ca501bb6e3\"}]},\"type\":\"ConnectorPlacement.EquallySpacedConnector\",\"uuid\":\"a3b713dd-1bd4-4226-93ff-27d7db6c05ec\"}],\"packageUris\":[\"http://schema.mathworks.com/mf0/Connector/R2020b\"],\"version\":\"1.0\"}"
  Bus Element Out1 : Outport  PortName=ROCC_DataBus

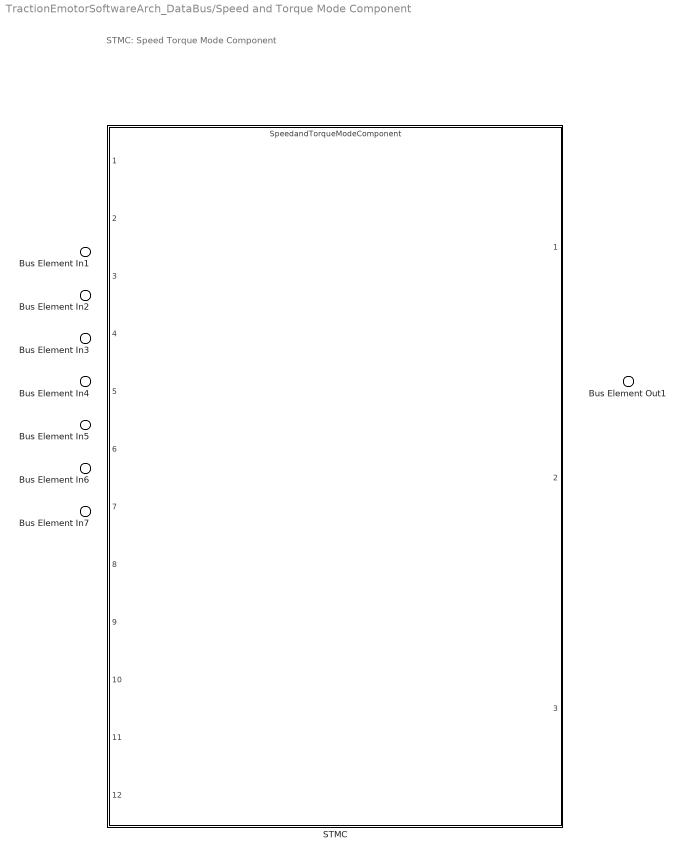
== system TractionEmotorSoftwareArch_DataBus/Speed and Torque Mode Component ==
  note: STMC: Speed Torque Mode Component
  Bus Element In1 : Inport  PortName=SMDC_DataBus
  Bus Element In2 : Inport  Port=2  PortName=CIDC_DataBus
  Bus Element In3 : Inport  Port=3  PortName=MFDC_DataBus
  Bus Element In4 : Inport  Port=4  PortName=PSCC_DataBus
  Bus Element In5 : Inport  Port=5  PortName=TDLC_DataBus
  Bus Element In6 : Inport  Port=6  PortName=TAEC_DataBus
  Bus Element In7 : Inport  Port=7  PortName=IHDC_DataBus
  STMC : ModelReference  ModelNameDialog=SpeedandTorqueModeComponent  SimulationMode=Normal  ScheduleRates=on  ModelReferenceVersion=7.0
      settings: PortSchema="{\"entries\":[{\"content\":{\"headerSize\":38,\"margin\":15,\"minimumSpacing\":25,\"sides\":[{\"content\":{\"connectorIds\":[\"In1\",\"In2\",\"In3\",\"In4\",\"In5\",\"In6\",\"In7\",\"In8\",\"In9\",\"In10\",\"In11\",\"In12\"]},\"type\":\"ConnectorPlacement.EquallySpacedRectSide\",\"uuid\":\"43f14977-22c5-403b-bcbc-53575b3aceee\"},{\"content\":{\"connectorIds\":[\"Out1\",\"Out2\",\"Out3\"],\"side\":\"RIGHT\"},\"type\":\"ConnectorPlacement.EquallySpacedRectSide\",\"uuid\":\"d93cf4b9-940c-436a-9f2b-9eb79a050f7a\"},{\"content\":{\"side\":\"TOP\"},\"type\":\"ConnectorPlacement.EquallySpacedRectSide\",\"uuid\":\"b3e7cb9e-f235-4106-b3bb-4ca948939197\"},{\"content\":{\"side\":\"HIDDEN\"},\"type\":\"ConnectorPlacement.EquallySpacedRectSide\",\"uuid\":\"94797063-f974-4ebd-b5aa-fa7798a2e67d\"}]},\"type\":\"ConnectorPlacement.EquallySpacedConnector\",\"uuid\":\"a3b713dd-1bd4-4226-93ff-27d7db6c05ec\"}],\"packageUris\":[\"http://schema.mathworks.com/mf0/Connector/R2020b\"],\"version\":\"1.0\"}"
  Bus Element Out1 : Outport  PortName=STMC_DataBus

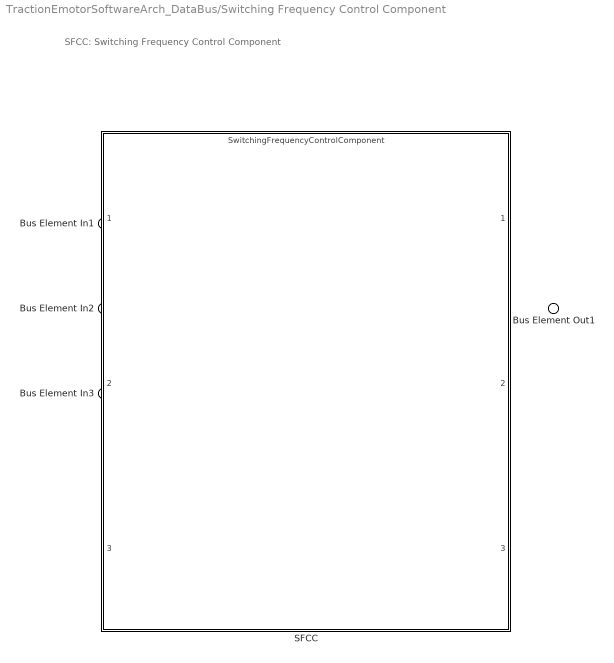
== system TractionEmotorSoftwareArch_DataBus/Switching Frequency Control Component ==
  note: SFCC: Switching Frequency Control Component
  Bus Element In1 : Inport  PortName=SMDC_DataBus
  Bus Element In2 : Inport  Port=2  PortName=PSCC_DataBus
  Bus Element In3 : Inport  Port=3  PortName=TDLC_DataBus
  SFCC : ModelReference  ModelNameDialog=SwitchingFrequencyControlComponent  SimulationMode=Normal  ScheduleRates=on  ModelReferenceVersion=7.0
      settings: PortSchema="{\"entries\":[{\"content\":{\"headerSize\":38,\"margin\":15,\"minimumSpacing\":25,\"sides\":[{\"content\":{\"connectorIds\":[\"In1\",\"In2\",\"In3\"]},\"type\":\"ConnectorPlacement.EquallySpacedRectSide\",\"uuid\":\"43f14977-22c5-403b-bcbc-53575b3aceee\"},{\"content\":{\"connectorIds\":[\"Out1\",\"Out2\",\"Out3\"],\"side\":\"RIGHT\"},\"type\":\"ConnectorPlacement.EquallySpacedRectSide\",\"uuid\":\"d93cf4b9-940c-436a-9f2b-9eb79a050f7a\"},{\"content\":{\"side\":\"TOP\"},\"type\":\"ConnectorPlacement.EquallySpacedRectSide\",\"uuid\":\"b3e7cb9e-f235-4106-b3bb-4ca948939197\"},{\"content\":{\"side\":\"HIDDEN\"},\"type\":\"ConnectorPlacement.EquallySpacedRectSide\",\"uuid\":\"9266f30c-a4d2-4de8-a7bf-3b429a5d927a\"}]},\"type\":\"ConnectorPlacement.EquallySpacedConnector\",\"uuid\":\"a3b713dd-1bd4-4226-93ff-27d7db6c05ec\"}],\"packageUris\":[\"http://schema.mathworks.com/mf0/Connector/R2020b\"],\"version\":\"1.0\"}"
  Bus Element Out1 : Outport  PortName=SFCC_DataBus

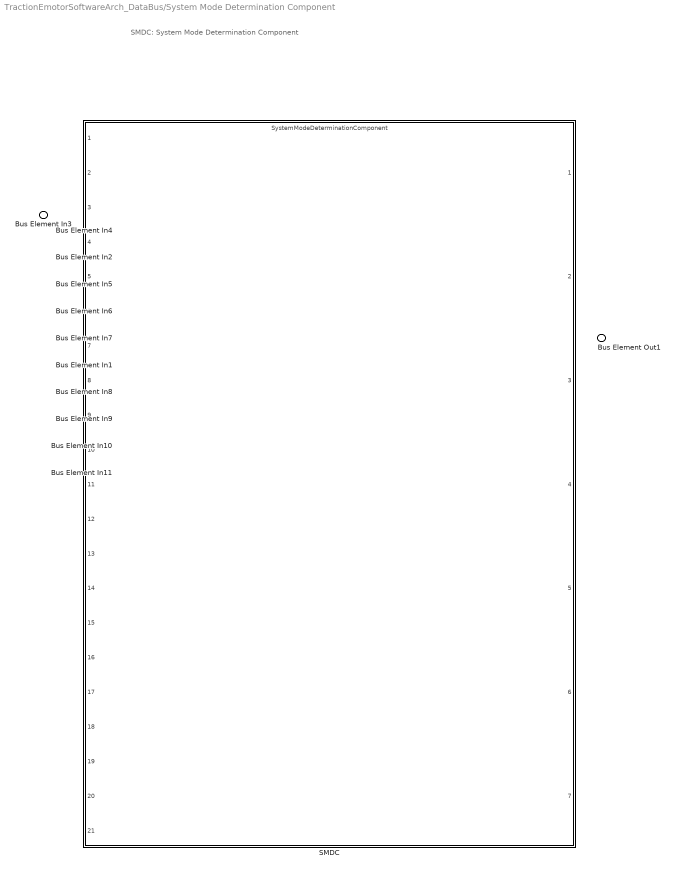
== system TractionEmotorSoftwareArch_DataBus/System Mode Determination Component  ==
  note: SMDC: System Mode Determination Component
  Bus Element In3 : Inport  PortName=CIDC_DataBus
  Bus Element In4 : Inport  Port=2  PortName=REDC_DataBus
  Bus Element In2 : Inport  Port=3  PortName=STDC_DataBus
  Bus Element In5 : Inport  Port=4  PortName=IHDC_DataBus
  Bus Element In6 : Inport  Port=5  PortName=MFDC_DataBus
  Bus Element In7 : Inport  Port=6  PortName=VSDC_DataBus
  Bus Element In1 : Inport  Port=7  PortName=ROCC_DataBus
  Bus Element In8 : Inport  Port=8  PortName=CSOC_DataBus
  Bus Element In9 : Inport  Port=9  PortName=VSOC_DataBus
  Bus Element In10 : Inport  Port=10  PortName=PSCC_DataBus
  Bus Element In11 : Inport  Port=11  PortName=STMC_DataBus
  SMDC : ModelReference  ModelNameDialog=SystemModeDeterminationComponent  SimulationMode=Normal  ScheduleRates=on  ModelReferenceVersion=7.0
      settings: PortSchema="{\"entries\":[{\"content\":{\"headerSize\":38,\"margin\":15,\"minimumSpacing\":25,\"sides\":[{\"content\":{\"connectorIds\":[\"In1\",\"In2\",\"In3\",\"In4\",\"In5\",\"In6\",\"In7\",\"In8\",\"In9\",\"In10\",\"In11\",\"In12\",\"In13\",\"In14\",\"In15\",\"In16\",\"In17\",\"In18\",\"In19\",\"In20\",\"In21\"]},\"type\":\"ConnectorPlacement.EquallySpacedRectSide\",\"uuid\":\"22c21561-7315-4f02-9846-f44950803b8a\"},{\"content\":{\"connectorIds\":[\"Out1\",\"Out2\",\"Out3\",\"Out4\",\"Out5\",\"Out6\",\"Out7\"],\"side\":\"RIGHT\"},\"type\":\"ConnectorPlacement.EquallySpacedRectSide\",\"uuid\":\"25f7ff13-02cc-4e6f-9448-3ba13ffa6ab9\"},{\"content\":{\"side\":\"TOP\"},\"type\":\"ConnectorPlacement.EquallySpacedRectSide\",\"uuid\":\"e3fd83fe-021a-4119-ab97-ca11ac661ffb\"},{\"content\":{\"side\":\"HIDDEN\"},\"type\":\"ConnectorPlacement.EquallySpacedRectSide\",\"uuid\":\"da59bf0e-3986-4578-a516-b8f6afbbd776\"}]},\"type\":\"ConnectorPlacement.EquallySpacedConnector\",\"uuid\":\"dc21257e-a83a-4628-a28d-2e2328c5c03a\"}],\"packageUris\":[\"http://schema.mathworks.com/mf0/Connector/R2020b\"],\"version\":\"1.0\"}"
  Bus Element Out1 : Outport  PortName=SMDC_DataBus

== system TractionEmotorSoftwareArch_DataBus/System Temperature Diagnostics Component ==
  note: STDC: System Temperature Diagnostics Component
  Bus Element In1 : Inport  PortName=CIDC_DataBus
  Bus Element In3 : Inport  Port=2  PortName=VSDC_DataBus
  Bus Element In2 : Inport  Port=3  PortName=STDC_faultStatus_Clear
  Bus Element Out5 : Outport  PortName=STDC_DataBus

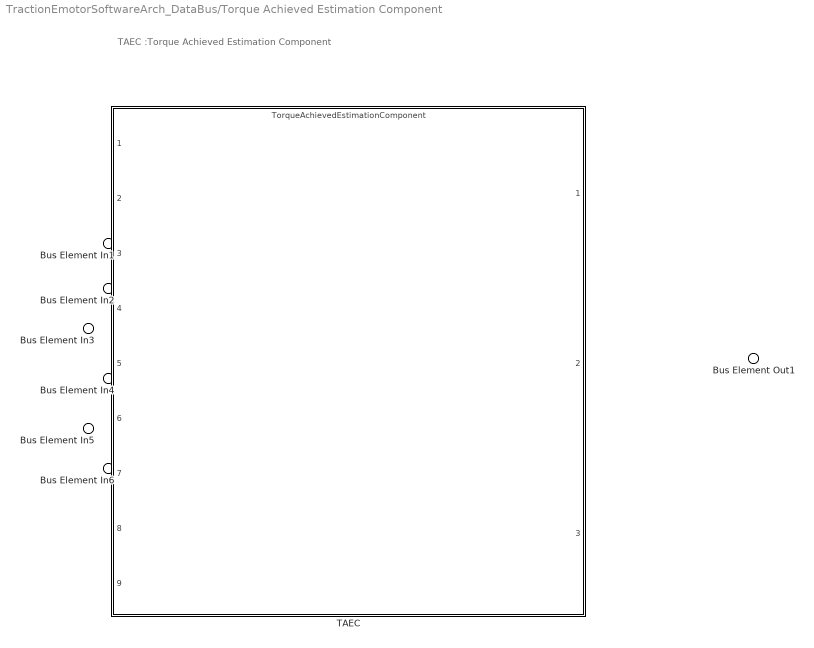
== system TractionEmotorSoftwareArch_DataBus/Torque Achieved Estimation Component ==
  note: TAEC :Torque Achieved Estimation Component
  Bus Element In1 : Inport  PortName=SMDC_DataBus
  Bus Element In2 : Inport  Port=2  PortName=CRFC_DataBus
  Bus Element In3 : Inport  Port=3  PortName=PWMC_DataBus
  Bus Element In4 : Inport  Port=4  PortName=IHDC_DataBus
  Bus Element In5 : Inport  Port=5  PortName=PSCC_DataBus
  Bus Element In6 : Inport  Port=6  PortName=STMC_DataBus
  TAEC : ModelReference  ModelNameDialog=TorqueAchievedEstimationComponent  SimulationMode=Normal  ScheduleRates=on  ModelReferenceVersion=8.1
      settings: PortSchema="{\"entries\":[{\"content\":{\"headerSize\":38,\"margin\":15,\"minimumSpacing\":25,\"sides\":[{\"content\":{\"connectorIds\":[\"In1\",\"In2\",\"In3\",\"In4\",\"In5\",\"In6\",\"In7\",\"In8\",\"In9\"]},\"type\":\"ConnectorPlacement.EquallySpacedRectSide\",\"uuid\":\"43f14977-22c5-403b-bcbc-53575b3aceee\"},{\"content\":{\"connectorIds\":[\"Out1\",\"Out2\",\"Out3\"],\"side\":\"RIGHT\"},\"type\":\"ConnectorPlacement.EquallySpacedRectSide\",\"uuid\":\"d93cf4b9-940c-436a-9f2b-9eb79a050f7a\"},{\"content\":{\"side\":\"TOP\"},\"type\":\"ConnectorPlacement.EquallySpacedRectSide\",\"uuid\":\"b3e7cb9e-f235-4106-b3bb-4ca948939197\"},{\"content\":{\"side\":\"HIDDEN\"},\"type\":\"ConnectorPlacement.EquallySpacedRectSide\",\"uuid\":\"a7ecf703-e5c1-483f-9530-0743023463c3\"}]},\"type\":\"ConnectorPlacement.EquallySpacedConnector\",\"uuid\":\"a3b713dd-1bd4-4226-93ff-27d7db6c05ec\"}],\"packageUris\":[\"http://schema.mathworks.com/mf0/Connector/R2020b\"],\"version\":\"1.0\"}"
  Bus Element Out1 : Outport  PortName=TAEC_DataBus

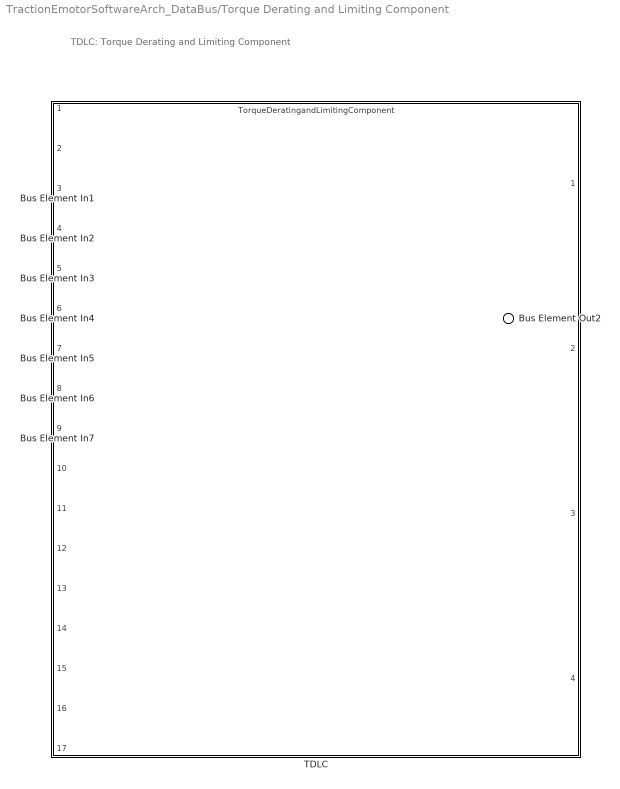
== system TractionEmotorSoftwareArch_DataBus/Torque Derating and Limiting Component ==
  note: TDLC: Torque Derating and Limiting Component
  Bus Element In1 : Inport  PortName=SMDC_DataBus
  Bus Element In2 : Inport  Port=2  PortName=DQRC_DataBus
  Bus Element In3 : Inport  Port=3  PortName=IHDC_DataBus
  Bus Element In4 : Inport  Port=4  PortName=PSCC_DataBus
  Bus Element In5 : Inport  Port=5  PortName=CIDC_DataBus
  Bus Element In6 : Inport  Port=6  PortName=STDC_DataBus
  Bus Element In7 : Inport  Port=7  PortName=STMC_DataBus
  TDLC : ModelReference  ModelNameDialog=TorqueDeratingandLimitingComponent  SimulationMode=Normal  ScheduleRates=on  ModelReferenceVersion=7.0
      settings: PortSchema="{\"entries\":[{\"content\":{\"headerSize\":38,\"margin\":15,\"minimumSpacing\":25,\"sides\":[{\"content\":{\"connectorIds\":[\"In1\",\"In2\",\"In3\",\"In4\",\"In5\",\"In6\",\"In7\",\"In8\",\"In9\",\"In10\",\"In11\",\"In12\",\"In13\",\"In14\",\"In15\",\"In16\",\"In17\"]},\"type\":\"ConnectorPlacement.EquallySpacedRectSide\",\"uuid\":\"43f14977-22c5-403b-bcbc-53575b3aceee\"},{\"content\":{\"connectorIds\":[\"Out1\",\"Out2\",\"Out3\",\"Out4\"],\"side\":\"RIGHT\"},\"type\":\"ConnectorPlacement.EquallySpacedRectSide\",\"uuid\":\"d93cf4b9-940c-436a-9f2b-9eb79a050f7a\"},{\"content\":{\"side\":\"TOP\"},\"type\":\"ConnectorPlacement.EquallySpacedRectSide\",\"uuid\":\"b3e7cb9e-f235-4106-b3bb-4ca948939197\"},{\"content\":{\"side\":\"HIDDEN\"},\"type\":\"ConnectorPlacement.EquallySpacedRectSide\",\"uuid\":\"20aa8750-7132-4faf-9c16-42c2f8fab151\"}]},\"type\":\"ConnectorPlacement.EquallySpacedConnector\",\"uuid\":\"a3b713dd-1bd4-4226-93ff-27d7db6c05ec\"}],\"packageUris\":[\"http://schema.mathworks.com/mf0/Connector/R2020b\"],\"version\":\"1.0\"}"
  Bus Element Out2 : Outport  PortName=TDLC_DataBus

== system TractionEmotorSoftwareArch_DataBus/Vehicle Status Diagnostics Component ==
  note: VSDC: Vehicle Status Diagnostics Component
  Bus Element Out8 : Outport  PortName=VSDC_DataBus

== system TractionEmotorSoftwareArch_DataBus/Voltage Sensor Offset Calibration Component ==
  note: VSOC: Voltage Sensor Offset Calibration Component
  Bus Element In1 : Inport  PortName=SMDC_DataBus
  Bus Element In2 : Inport  Port=2  PortName=CIDC_DataBus
  Bus Element In3 : Inport  Port=3  PortName=IHDC_DataBus
  VSOC : ModelReference  ModelNameDialog=VoltageSensorOffsetCalibrationComponent  SimulationMode=Normal  ScheduleRates=on  ModelReferenceVersion=7.0
      settings: PortSchema="{\"entries\":[{\"content\":{\"headerSize\":38,\"margin\":15,\"minimumSpacing\":25,\"sides\":[{\"content\":{\"connectorIds\":[\"In1\",\"In2\",\"In3\"]},\"type\":\"ConnectorPlacement.EquallySpacedRectSide\",\"uuid\":\"43f14977-22c5-403b-bcbc-53575b3aceee\"},{\"content\":{\"connectorIds\":[\"Out1\",\"Out2\",\"Out3\",\"Out4\"],\"side\":\"RIGHT\"},\"type\":\"ConnectorPlacement.EquallySpacedRectSide\",\"uuid\":\"d93cf4b9-940c-436a-9f2b-9eb79a050f7a\"},{\"content\":{\"side\":\"TOP\"},\"type\":\"ConnectorPlacement.EquallySpacedRectSide\",\"uuid\":\"b3e7cb9e-f235-4106-b3bb-4ca948939197\"},{\"content\":{\"side\":\"HIDDEN\"},\"type\":\"ConnectorPlacement.EquallySpacedRectSide\",\"uuid\":\"dbd5cbf7-ab36-4124-a1e3-d8ae42d9bf1c\"}]},\"type\":\"ConnectorPlacement.EquallySpacedConnector\",\"uuid\":\"a3b713dd-1bd4-4226-93ff-27d7db6c05ec\"}],\"packageUris\":[\"http://schema.mathworks.com/mf0/Connector/R2020b\"],\"version\":\"1.0\"}"
  Bus Element Out1 : Outport  PortName=VSOC_DataBus
